simulink model "test1_5_org"  (Simulink 10.0)
settings: Solver=ode45  StartTime=0.0  StopTime=10.0  RelTol=1e-3  EnableMultiTasking=on
settings Model: Creator=asus  LastModifiedBy=bhisma
settings DataIOCC: LimitDataPoints=on
settings DebuggingCC: UnderspecifiedInitializationDetection=Simplified  MergeDetectMultiDrivingBlocksExec=error  SolverPrmCheckMsg=warning
settings GRTTargetCC: GeneratePreprocessorConditionals=Disable all  CombineOutputUpdateFcns=on  GRTInterface=off
settings ConfigComp: CovExternalEMLEnable=off  CovSFcnEnable=off

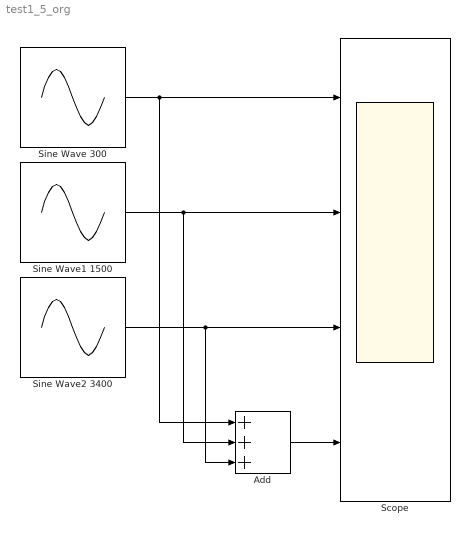
== system test1_5_org ==
  Add : Sum  Inputs=+++
  Scope : Scope  NumInputPorts=4
  Sine Wave 300 : Sin  Amplitude=0.3  Frequency=300  SampleTime=1/8000
  Sine Wave1 1500 : Sin  Frequency=1500  SampleTime=1/8000
  Sine Wave2 3400 : Sin  Amplitude=0.3  Frequency=3400  SampleTime=1/8000
  wires:
  Sine Wave 300/1 -> Scope/1, Add/1
  Sine Wave1 1500/1 -> Scope/2, Add/2
  Sine Wave2 3400/1 -> Add/3, Scope/3
  Add/1 -> Scope/4
